simulink model "EvPowertrainController3EMDualRear"  (R2025b)
settings: configuration reference "VehicleFixed10ms" (kept outside this file)
model workspace (MAT data in the model file):
  CtrlVcuAccelPdlBpts = [0 0.8 1]
  CtrlVcuBattPnlty = 10000000
  CtrlVcuBattSOCBpts = [0 20 60 80 100]
  CtrlVcuCnstrntPnltyFctr = 10000000
  CtrlVcuEMPnlty = 100
  CtrlVcuEMTrqSplitGrid = 200
  CtrlVcuFallRate = -500
  CtrlVcuMaxAccelG = 1
  CtrlVcuMaxDecelG = -1.5
  CtrlVcuPwrDeltaPnlty = 50
  CtrlVcuPwrRatePnlty = [25 25 100]
  CtrlVcuRiseRate = 500
  CtrlVcuRoadMuEst = 0.8
  CtrlVcuSftyFctr = 0.9
  CtrlVcuTracPwrErrPnlty = 25
  CtrlVcuTrqVecBrkThresh = 0.01
  CtrlVcuTrqVecIGain = 0
  CtrlVcuTrqVecMinTrq = 25
  CtrlVcuTrqVecPGain = -2000
  CtrlVcuTrqVecSteerThresh = 0.349065850399
  CtrlVcuTrqVecVelThresh = 2.5
  N_P0 = 3
undefined symbols (not defined in the file): CtrlBcuTrlrBrkGain, CtrlVcuEvChrgLmtBpt, CtrlVcuEvRegenBrkCutOff, CtrlVcuEvRegenBrkSpdBpt, CtrlVcuEvSocBpt, eff, EnvGrvty, PlntBrkActrBoreFrnt, PlntBrkActrBoreRear, PlntBrkFrntBias, PlntBrkKinFricCffFrnt, PlntBrkKinFricCffRear, PlntBrkNumPadsFrnt, PlntBrkNumPadsRear, PlntBrkPadMeanRadiusFrnt, PlntBrkPadMeanRadiusRear, PlntBrkPrsFctr, PlntBrkRearBias, PlntDiffrntl2Eff, PlntDiffrntl2Ratio, PlntDiffrntlEff, PlntDiffrntlRatio, PlntEM1EffTbl, PlntEM1Spd, PlntEM1SpdEff, PlntEM1TransEff, PlntEM1TransGearRatio, PlntEM1Trq, PlntEM1TrqEff, PlntEM2EffTbl, PlntEM2Spd, PlntEM2SpdEff, PlntEM2TransEff, PlntEM2TransGearRatio, PlntEM2Trq, PlntEM2TrqEff, PlntEM3EffTbl, PlntEM3Spd, PlntEM3SpdEff, PlntEM3TransEff, PlntEM3TransGearRatio, PlntEM3Trq, PlntEM3TrqEff, PlntEMWhlGearEffFL, PlntEMWhlGearEffRL, PlntEMWhlGearRatioFL, PlntEMWhlGearRatioRL, PlntTransEffSpdBpt, PlntTransEffTbl, PlntTransEffTempBpt, PlntTransEffTrqBpt, PlntTransGearNumVect, PlntTransGearRatioVect, PlntVehCGHgtAxl, PlntVehDstCGFrntAxl, PlntVehDstCGRearAxl, PlntVehMass, PlntWhlLdRadiusFrnt, PlntWhlLdRadiusRear
libraries: simulink x16, autolibutils x2, slpidlib x2
(part 4 of 5)

== system EvPowertrainController3EMDualRear/Energy Management/Calculate Average EMSpd and Wheel Torque Curves for Front and Rear Axles/3EM Dual Rear/EMTrq2WhlTrqRear/Single Speed Transmission ==
  EMTrqCmd : Inport
  EMSpd : Inport  Port=2
  Divide2 : Product  Inputs=**
  Dual EMs : Gain  Gain=2
  Gain3 : Gain  Gain=PlntEMWhlGearRatioRL*PlntEM2TransGearRatio
  Gear Eta : Subsystem
  WhlMotTrq : Outport  VectorParamsAs1DForOutWhenUnconnected=off
  wires:
  Gear Eta/1(eta) -> Divide2/1
  EMTrqCmd/1 -> Dual EMs/1
  EMSpd/1 -> Gear Eta/1(SpdIn)
  Divide2/1 -> WhlMotTrq/1
  Gain3/1 -> Divide2/2
  Dual EMs/1 -> Gain3/1, Gear Eta/2(TrqIn)

== system EvPowertrainController3EMDualRear/Energy Management/Calculate Average EMSpd and Wheel Torque Curves for Front and Rear Axles/3EM Dual Rear/EMTrq2WhlTrqRear/Transmission ==
  Gear : Inport
  EMTrqCmd : Inport  Port=2
  EMSpd : Inport  Port=3
  Diff Eta : Subsystem
  Divide : Product  Inputs=**
  Divide1 : Product  Inputs=**
  Divide2 : Product  Inputs=**
  Divide3 : Product  Inputs=*/
  Gain : Gain  Gain=PlntDiffrntl2Ratio
  Gear ratio look up : LookupNDDirect  NumberOfTableDimensions=1  Table=PlntTransGearRatioVect
  Trans Eta : Subsystem
  WhlMotTrq : Outport  VectorParamsAs1DForOutWhenUnconnected=off
  wires:
  EMSpd/1 -> Trans Eta/2(SpdIn), [Spd]
  EMTrqCmd/1 -> Trans Eta/1(TrqIn), Divide/2
  Divide3/1 -> Diff Eta/1(SpdIn)
  [Spd] -> Divide3/1
  Diff Eta/1(eta) -> Divide2/1
  Divide2/1 -> WhlMotTrq/1
  Divide1/1 -> Gain/1, Diff Eta/2(TrqIn)
  Trans Eta/1(eta) -> Divide1/1
  Gear/1 -> Gear ratio look up/1, Trans Eta/3(Gear)
  Divide/1 -> Divide1/2
  Gear ratio look up/1 -> Divide/1, Divide3/2
  Gain/1 -> Divide2/2

== system EvPowertrainController3EMDualRear/Energy Management/Calculate Average EMSpd and Wheel Torque Curves for Front and Rear Axles/4EM/EMTrq2WhlTrqFrnt/Single Speed Transmission ==
  EMTrqCmd : Inport
  EMSpd : Inport  Port=2
  Divide2 : Product  Inputs=**
  Dual EMs : Gain  Gain=2
  Gain3 : Gain  Gain=PlntEMWhlGearRatioFL*PlntEM1TransGearRatio
  Gear Eta : Subsystem
  WhlMotTrq : Outport  VectorParamsAs1DForOutWhenUnconnected=off
  wires:
  Gain3/1 -> Divide2/2
  Divide2/1 -> WhlMotTrq/1
  EMSpd/1 -> Gear Eta/1(SpdIn)
  EMTrqCmd/1 -> Dual EMs/1
  Gear Eta/1(eta) -> Divide2/1
  Dual EMs/1 -> Gear Eta/2(TrqIn), Gain3/1

== system EvPowertrainController3EMDualRear/Energy Management/Calculate Average EMSpd and Wheel Torque Curves for Front and Rear Axles/4EM/EMTrq2WhlTrqFrnt/Transmission ==
  Gear : Inport
  EMTrqCmd : Inport  Port=2
  EMSpd : Inport  Port=3
  Diff Eta : Subsystem
  Divide : Product  Inputs=**
  Divide1 : Product  Inputs=**
  Divide2 : Product  Inputs=**
  Divide3 : Product  Inputs=*/
  Gain : Gain  Gain=PlntDiffrntlRatio
  Gear ratio look up : LookupNDDirect  NumberOfTableDimensions=1  Table=PlntTransGearRatioVect
  Trans Eta : Subsystem
  WhlMotTrq : Outport  VectorParamsAs1DForOutWhenUnconnected=off
  wires:
  EMSpd/1 -> Trans Eta/2(SpdIn), [Spd]
  EMTrqCmd/1 -> Trans Eta/1(TrqIn), Divide/2
  Divide3/1 -> Diff Eta/1(SpdIn)
  [Spd] -> Divide3/1
  Diff Eta/1(eta) -> Divide2/1
  Divide2/1 -> WhlMotTrq/1
  Divide1/1 -> Gain/1, Diff Eta/2(TrqIn)
  Trans Eta/1(eta) -> Divide1/1
  Gear/1 -> Gear ratio look up/1, Trans Eta/3(Gear)
  Divide/1 -> Divide1/2
  Gear ratio look up/1 -> Divide/1, Divide3/2
  Gain/1 -> Divide2/2

== system EvPowertrainController3EMDualRear/Energy Management/Calculate Average EMSpd and Wheel Torque Curves for Front and Rear Axles/4EM/EMTrq2WhlTrqRear/Single Speed Transmission ==
  EMTrqCmd : Inport
  EMSpd : Inport  Port=2
  Divide2 : Product  Inputs=**
  Dual EMs : Gain  Gain=2
  Gain3 : Gain  Gain=PlntEMWhlGearRatioRL*PlntEM3TransGearRatio
  Gear Eta : Subsystem
  WhlMotTrq : Outport  VectorParamsAs1DForOutWhenUnconnected=off
  wires:
  Gain3/1 -> Divide2/2
  Divide2/1 -> WhlMotTrq/1
  EMSpd/1 -> Gear Eta/1(SpdIn)
  EMTrqCmd/1 -> Dual EMs/1
  Gear Eta/1(eta) -> Divide2/1
  Dual EMs/1 -> Gear Eta/2(TrqIn), Gain3/1

== system EvPowertrainController3EMDualRear/Energy Management/Calculate Average EMSpd and Wheel Torque Curves for Front and Rear Axles/4EM/EMTrq2WhlTrqRear/Transmission ==
  Gear : Inport
  EMTrqCmd : Inport  Port=2
  EMSpd : Inport  Port=3
  Diff Eta : Subsystem
  Divide : Product  Inputs=**
  Divide1 : Product  Inputs=**
  Divide2 : Product  Inputs=**
  Divide3 : Product  Inputs=*/
  Gain : Gain  Gain=PlntDiffrntl2Ratio
  Gear ratio look up : LookupNDDirect  NumberOfTableDimensions=1  Table=PlntTransGearRatioVect
  Trans Eta : Subsystem
  WhlMotTrq : Outport  VectorParamsAs1DForOutWhenUnconnected=off
  wires:
  Gain/1 -> Divide2/2
  Gear ratio look up/1 -> Divide3/2, Divide/1
  Divide/1 -> Divide1/2
  Gear/1 -> Trans Eta/3(Gear), Gear ratio look up/1
  Trans Eta/1(eta) -> Divide1/1
  Divide1/1 -> Diff Eta/2(TrqIn), Gain/1
  Divide2/1 -> WhlMotTrq/1
  Diff Eta/1(eta) -> Divide2/1
  [Spd] -> Divide3/1
  Divide3/1 -> Diff Eta/1(SpdIn)
  EMTrqCmd/1 -> Divide/2, Trans Eta/1(TrqIn)
  EMSpd/1 -> [Spd], Trans Eta/2(SpdIn)

== system EvPowertrainController3EMDualRear/Energy Management/Control Domain /Front Axle EM Torque Vector/2EM or 3EM Dual Rear/Diff Eta ==
  note: Pwr >= 0, v = 1
      | Pwr < 0, v= -1
  SpdIn : Inport
  TrqIn : Inport  Port=2
  Constant : Constant  Value=PlntDiffrntlEff*PlntEM1TransEff
  Constant1 : Constant  SampleTime=-1
  Constant2 : Constant  Value=-1  SampleTime=-1
  Math Function1 : Math  Operator=pow  SignedPower=on  OutputSignalType=real
  Product1 : Product
  Switch2 : Switch  SaturateOnIntegerOverflow=off  InputSameDT=off
  eta : Outport  VectorParamsAs1DForOutWhenUnconnected=off
  wires:
  TrqIn/1 -> Product1/1
  Math Function1/1 -> eta/1
  Switch2/1 -> Math Function1/2
  Product1/1 -> Switch2/2
  Constant1/1 -> Switch2/1
  Constant2/1 -> Switch2/3
  Constant/1 -> Math Function1/1
  SpdIn/1 -> Product1/2

== system EvPowertrainController3EMDualRear/Energy Management/Control Domain /Front Axle EM Torque Vector/3EM Dual Front or 4EM/Gear Eta ==
  note: Pwr >= 0, v = 1
      | Pwr < 0, v= -1
  SpdIn : Inport
  TrqIn : Inport  Port=2
  Constant : Constant  Value=PlntEMWhlGearEffFL*PlntEM1TransEff
  Constant1 : Constant  SampleTime=-1
  Constant2 : Constant  Value=-1  SampleTime=-1
  Math Function1 : Math  Operator=pow  SignedPower=on  OutputSignalType=real
  Product1 : Product
  Switch2 : Switch  SaturateOnIntegerOverflow=off  InputSameDT=off
  eta : Outport  VectorParamsAs1DForOutWhenUnconnected=off
  wires:
  TrqIn/1 -> Product1/1
  Math Function1/1 -> eta/1
  Switch2/1 -> Math Function1/2
  Product1/1 -> Switch2/2
  Constant1/1 -> Switch2/1
  Constant2/1 -> Switch2/3
  Constant/1 -> Math Function1/1
  SpdIn/1 -> Product1/2

== system EvPowertrainController3EMDualRear/Energy Management/Control Domain /Rear Axle EM Torque Vector/2EM/Diff Eta ==
  note: Pwr >= 0, v = 1
      | Pwr < 0, v= -1
  SpdIn : Inport
  TrqIn : Inport  Port=2
  Constant : Constant  Value=PlntDiffrntl2Eff*PlntEM2TransEff
  Constant1 : Constant  SampleTime=-1
  Constant2 : Constant  Value=-1  SampleTime=-1
  Math Function1 : Math  Operator=pow  SignedPower=on  OutputSignalType=real
  Product1 : Product
  Switch2 : Switch  SaturateOnIntegerOverflow=off  InputSameDT=off
  eta : Outport  VectorParamsAs1DForOutWhenUnconnected=off
  wires:
  SpdIn/1 -> Product1/2
  Constant/1 -> Math Function1/1
  Constant2/1 -> Switch2/3
  Constant1/1 -> Switch2/1
  Product1/1 -> Switch2/2
  Switch2/1 -> Math Function1/2
  Math Function1/1 -> eta/1
  TrqIn/1 -> Product1/1

== system EvPowertrainController3EMDualRear/Energy Management/Control Domain /Rear Axle EM Torque Vector/3EM Dual Front/Diff Eta ==
  note: Pwr >= 0, v = 1
      | Pwr < 0, v= -1
  SpdIn : Inport
  TrqIn : Inport  Port=2
  Constant : Constant  Value=PlntDiffrntl2Eff*PlntEM3TransEff
  Constant1 : Constant  SampleTime=-1
  Constant2 : Constant  Value=-1  SampleTime=-1
  Math Function1 : Math  Operator=pow  SignedPower=on  OutputSignalType=real
  Product1 : Product
  Switch2 : Switch  SaturateOnIntegerOverflow=off  InputSameDT=off
  eta : Outport  VectorParamsAs1DForOutWhenUnconnected=off
  wires:
  TrqIn/1 -> Product1/1
  Math Function1/1 -> eta/1
  Switch2/1 -> Math Function1/2
  Product1/1 -> Switch2/2
  Constant1/1 -> Switch2/1
  Constant2/1 -> Switch2/3
  Constant/1 -> Math Function1/1
  SpdIn/1 -> Product1/2

== system EvPowertrainController3EMDualRear/Energy Management/Control Domain /Rear Axle EM Torque Vector/3EM Dual Rear or 4EM/Gear Eta ==
  note: Pwr >= 0, v = 1
      | Pwr < 0, v= -1
  SpdIn : Inport
  TrqIn : Inport  Port=2
  Constant : Constant  Value=PlntEMWhlGearEffRL*PlntEM3TransEff
  Constant1 : Constant  SampleTime=-1
  Constant2 : Constant  Value=-1  SampleTime=-1
  Math Function1 : Math  Operator=pow  SignedPower=on  OutputSignalType=real
  Product1 : Product
  Switch2 : Switch  SaturateOnIntegerOverflow=off  InputSameDT=off
  eta : Outport  VectorParamsAs1DForOutWhenUnconnected=off
  wires:
  SpdIn/1 -> Product1/2
  Constant/1 -> Math Function1/1
  Constant2/1 -> Switch2/3
  Constant1/1 -> Switch2/1
  Product1/1 -> Switch2/2
  Switch2/1 -> Math Function1/2
  Math Function1/1 -> eta/1
  TrqIn/1 -> Product1/1

== system EvPowertrainController3EMDualRear/Energy Management/Powertrain Constraints /Battery Constraint/Electrical Current/DC-DC Eta ==
  In : Inport
  DC-DC Eta : Subsystem  VariantControl=1
  No DC-DC : Subsystem  VariantControl=0
  Out : Outport  VectorParamsAs1DForOutWhenUnconnected=off

== system EvPowertrainController3EMDualRear/Energy Management/Powertrain Constraints /EM Constraint Front/Tabular Power Loss Data/2EM or 3EM Dual Rear ==
  note: Pelec_req = Pmech_req*Eff^k,
      | k = -1 if Motoring >= 0,
      | k = 1 if Generating < 0
  note: Check if Motoring
      | or Generating
  EMAvgSpdVec : Inport
  WhlEMTrqSatVec : Inport  Port=2
  Abs : Abs  SaturateOnIntegerOverflow=off
  Abs1 : Abs  SaturateOnIntegerOverflow=off
  Constant1 : Constant  Value=-1  SampleTime=-1
  Constant2 : Constant  SampleTime=-1
  Eff Map : Lookup_n-D  BreakpointsForDimension1=PlntEM1SpdEff  BreakpointsForDimension2=PlntEM1TrqEff  BeginIndexSearchUsingPreviousIndexResult=on  Table=PlntEM1EffTbl  ExtrapMethod=Clip  UseLastTableValue=on  InternalRulePriority=Speed  OutDataTypeStr=Inherit: Inherit from 'Table data'  RndMeth=Simplest
      settings: InputPortMap=u0,u1
  Gain2 : Gain  Gain=1/100
  Math Function1 : Math  Operator=pow  SignedPower=on  OutputSignalType=real
  Product1 : Product
  Product4 : Product
  Switch2 : Switch  SaturateOnIntegerOverflow=off  InputSameDT=off
  WhlTrq2EMTrq : Subsystem  VariantControl=2EM or 3EMDualFront
  EMPwrElecVec : Outport  VectorParamsAs1DForOutWhenUnconnected=off
  wires:
  WhlEMTrqSatVec/1 -> WhlTrq2EMTrq/2(WhlTrqCmd)
  EMAvgSpdVec/1 -> WhlTrq2EMTrq/1(EMSpd), Product1/1, Abs/1
  Eff Map/1 -> Gain2/1
  Abs1/1 -> Eff Map/2
  Abs/1 -> Eff Map/1
  Gain2/1 -> Math Function1/1
  Constant2/1 -> Switch2/3
  Constant1/1 -> Switch2/1
  Product1/1 -> Switch2/2, Product4/1
  Switch2/1 -> Math Function1/2
  Math Function1/1 -> Product4/2
  Product4/1 -> EMPwrElecVec/1
  WhlTrq2EMTrq/1(EMTrq) -> Abs1/1, Product1/2

== system EvPowertrainController3EMDualRear/Energy Management/Powertrain Constraints /EM Constraint Front/Tabular Power Loss Data/3EM Dual Front or 4EM ==
  note: Check if Motoring
      | or Generating
  note: Pelec_req = Pmech_req*Eff^k,
      | k = -1 if Motoring >= 0,
      | k = 1 if Generating < 0
  EMAvgSpdVec : Inport
  WhlEMTrqSatVec : Inport  Port=2
  Abs : Abs  SaturateOnIntegerOverflow=off
  Abs1 : Abs  SaturateOnIntegerOverflow=off
  Constant1 : Constant  Value=-1  SampleTime=-1
  Constant2 : Constant  SampleTime=-1
  Dual EMs : Gain  Gain=2
  Eff Map : Lookup_n-D  BreakpointsForDimension1=PlntEM1SpdEff  BreakpointsForDimension2=PlntEM1TrqEff  BeginIndexSearchUsingPreviousIndexResult=on  Table=PlntEM1EffTbl  ExtrapMethod=Clip  UseLastTableValue=on  InternalRulePriority=Speed  OutDataTypeStr=Inherit: Inherit from 'Table data'  RndMeth=Simplest
      settings: InputPortMap=u0,u1
  Gain2 : Gain  Gain=1/100
  Math Function1 : Math  Operator=pow  SignedPower=on  OutputSignalType=real
  Product1 : Product
  Product4 : Product
  Switch2 : Switch  SaturateOnIntegerOverflow=off  InputSameDT=off
  WhlTrq2EMTrq : Subsystem  VariantControl=3EMDualRear or 4EM
  EMPwrElecVec : Outport  VectorParamsAs1DForOutWhenUnconnected=off
  wires:
  WhlTrq2EMTrq/1(EMTrq) -> Product1/2, Abs1/1
  Product4/1 -> Dual EMs/1
  Math Function1/1 -> Product4/2
  Switch2/1 -> Math Function1/2
  Product1/1 -> Product4/1, Switch2/2
  Constant1/1 -> Switch2/1
  Constant2/1 -> Switch2/3
  Gain2/1 -> Math Function1/1
  Abs/1 -> Eff Map/1
  Abs1/1 -> Eff Map/2
  Eff Map/1 -> Gain2/1
  EMAvgSpdVec/1 -> WhlTrq2EMTrq/1(EMSpd), Abs/1, Product1/1
  WhlEMTrqSatVec/1 -> WhlTrq2EMTrq/2(WhlTrqCmd)
  Dual EMs/1 -> EMPwrElecVec/1

== system EvPowertrainController3EMDualRear/Energy Management/Powertrain Constraints /EM Constraint Front/Wheel Torque Saturation for Max g Rates/Wheel Torque Limit at Max g Rates ==
  note: Braking sign convention
  Constant6 : Constant  Value=CtrlVcuMaxDecelG  SampleTime=-1
  Constant7 : Constant  Value=CtrlVcuMaxAccelG  SampleTime=-1
  Gain : Gain  Gain=-1
  Wheel Torque at Max Acceleration Rate : Subsystem  VariantControl=tractorVariant==3
  Wheel Torque at Max Deceleration Rate : Subsystem  VariantControl=tractorVariant==3
  WhlTrqLmt_Accel : Outport
  WhlTrqLmt_Brk : Outport  Port=2
  wires:
  Constant6/1 -> Wheel Torque at Max Deceleration Rate/1(MaxAcc)
  Constant7/1 -> Wheel Torque at Max Acceleration Rate/1(MaxAcc)
  Wheel Torque at Max Acceleration Rate/1(WhlTrqLmt) -> WhlTrqLmt_Accel/1
  Wheel Torque at Max Deceleration Rate/1(WhlTrqLmt) -> Gain/1
  Gain/1 -> WhlTrqLmt_Brk/1

== system EvPowertrainController3EMDualRear/Energy Management/Powertrain Constraints /EM Constraint Rear/Tabular Power Loss Data/2EM ==
  note: Pelec_req = Pmech_req*Eff^k,
      | k = -1 if Motoring >= 0,
      | k = 1 if Generating < 0
  note: Check if Motoring
      | or Generating
  EMAvgSpdVec : Inport
  WhlEMTrqSatVec : Inport  Port=2
  Abs : Abs  SaturateOnIntegerOverflow=off
  Abs1 : Abs  SaturateOnIntegerOverflow=off
  Constant1 : Constant  Value=-1  SampleTime=-1
  Constant2 : Constant  SampleTime=-1
  Eff Map : Lookup_n-D  BreakpointsForDimension1=PlntEM2SpdEff  BreakpointsForDimension2=PlntEM2TrqEff  BeginIndexSearchUsingPreviousIndexResult=on  Table=PlntEM2EffTbl  ExtrapMethod=Clip  UseLastTableValue=on  InternalRulePriority=Speed  OutDataTypeStr=Inherit: Inherit from 'Table data'  RndMeth=Simplest
      settings: InputPortMap=u0,u1
  Gain2 : Gain  Gain=1/100
  Math Function1 : Math  Operator=pow  SignedPower=on  OutputSignalType=real
  Product1 : Product
  Product4 : Product
  Switch2 : Switch  SaturateOnIntegerOverflow=off  InputSameDT=off
  WhlTrq2EMTrq : Subsystem  VariantControl=2EM or 3EMDualFront
  EMPwrElecVec : Outport  VectorParamsAs1DForOutWhenUnconnected=off
  wires:
  WhlEMTrqSatVec/1 -> WhlTrq2EMTrq/2(WhlTrqCmd)
  EMAvgSpdVec/1 -> WhlTrq2EMTrq/1(EMSpd), Product1/1, Abs/1
  Eff Map/1 -> Gain2/1
  Abs1/1 -> Eff Map/2
  Abs/1 -> Eff Map/1
  Gain2/1 -> Math Function1/1
  Constant2/1 -> Switch2/3
  Constant1/1 -> Switch2/1
  Product1/1 -> Switch2/2, Product4/1
  Switch2/1 -> Math Function1/2
  Math Function1/1 -> Product4/2
  Product4/1 -> EMPwrElecVec/1
  WhlTrq2EMTrq/1(EMTrq) -> Abs1/1, Product1/2

== system EvPowertrainController3EMDualRear/Energy Management/Powertrain Constraints /EM Constraint Rear/Tabular Power Loss Data/3EM Dual Front ==
  note: Check if Motoring
      | or Generating
  note: Pelec_req = Pmech_req*Eff^k,
      | k = -1 if Motoring >= 0,
      | k = 1 if Generating < 0
  EMAvgSpdVec : Inport
  WhlEMTrqSatVec : Inport  Port=2
  Abs : Abs  SaturateOnIntegerOverflow=off
  Abs1 : Abs  SaturateOnIntegerOverflow=off
  Constant1 : Constant  Value=-1  SampleTime=-1
  Constant2 : Constant  SampleTime=-1
  Eff Map : Lookup_n-D  BreakpointsForDimension1=PlntEM3SpdEff  BreakpointsForDimension2=PlntEM3TrqEff  BeginIndexSearchUsingPreviousIndexResult=on  Table=PlntEM3EffTbl  ExtrapMethod=Clip  UseLastTableValue=on  InternalRulePriority=Speed  OutDataTypeStr=Inherit: Inherit from 'Table data'  RndMeth=Simplest
      settings: InputPortMap=u0,u1
  Gain2 : Gain  Gain=1/100
  Math Function1 : Math  Operator=pow  SignedPower=on  OutputSignalType=real
  Product1 : Product
  Product4 : Product
  Switch2 : Switch  SaturateOnIntegerOverflow=off  InputSameDT=off
  WhlTrq2EMTrq : Subsystem  VariantControl=2EM or 3EMDualFront
  EMPwrElecVec : Outport  VectorParamsAs1DForOutWhenUnconnected=off
  wires:
  WhlTrq2EMTrq/1(EMTrq) -> Product1/2, Abs1/1
  Product4/1 -> EMPwrElecVec/1
  Math Function1/1 -> Product4/2
  Switch2/1 -> Math Function1/2
  Product1/1 -> Product4/1, Switch2/2
  Constant1/1 -> Switch2/1
  Constant2/1 -> Switch2/3
  Gain2/1 -> Math Function1/1
  Abs/1 -> Eff Map/1
  Abs1/1 -> Eff Map/2
  Eff Map/1 -> Gain2/1
  EMAvgSpdVec/1 -> Abs/1, Product1/1, WhlTrq2EMTrq/1(EMSpd)
  WhlEMTrqSatVec/1 -> WhlTrq2EMTrq/2(WhlTrqCmd)

== system EvPowertrainController3EMDualRear/Energy Management/Powertrain Constraints /EM Constraint Rear/Tabular Power Loss Data/3EM Dual Rear or 4EM ==
  note: Check if Motoring
      | or Generating
  note: Pelec_req = Pmech_req*Eff^k,
      | k = -1 if Motoring >= 0,
      | k = 1 if Generating < 0
  EMAvgSpdVec : Inport
  WhlEMTrqSatVec : Inport  Port=2
  Abs : Abs  SaturateOnIntegerOverflow=off
  Abs1 : Abs  SaturateOnIntegerOverflow=off
  Constant1 : Constant  Value=-1  SampleTime=-1
  Constant2 : Constant  SampleTime=-1
  Dual EMs : Gain  Gain=2
  Eff Map : Lookup_n-D  BreakpointsForDimension1=PlntEM3SpdEff  BreakpointsForDimension2=PlntEM3TrqEff  BeginIndexSearchUsingPreviousIndexResult=on  Table=PlntEM3EffTbl  ExtrapMethod=Clip  UseLastTableValue=on  InternalRulePriority=Speed  OutDataTypeStr=Inherit: Inherit from 'Table data'  RndMeth=Simplest
      settings: InputPortMap=u0,u1
  Gain2 : Gain  Gain=1/100
  Math Function1 : Math  Operator=pow  SignedPower=on  OutputSignalType=real
  Product1 : Product
  Product4 : Product
  Switch2 : Switch  SaturateOnIntegerOverflow=off  InputSameDT=off
  WhlTrq2EMTrq : Subsystem  VariantControl=3EMDualRear or 4EM
  EMPwrElecVec : Outport  VectorParamsAs1DForOutWhenUnconnected=off
  wires:
  WhlTrq2EMTrq/1(EMTrq) -> Product1/2, Abs1/1
  Product4/1 -> Dual EMs/1
  Math Function1/1 -> Product4/2
  Switch2/1 -> Math Function1/2
  Product1/1 -> Product4/1, Switch2/2
  Constant1/1 -> Switch2/1
  Constant2/1 -> Switch2/3
  Gain2/1 -> Math Function1/1
  Abs/1 -> Eff Map/1
  Abs1/1 -> Eff Map/2
  Eff Map/1 -> Gain2/1
  EMAvgSpdVec/1 -> WhlTrq2EMTrq/1(EMSpd), Abs/1, Product1/1
  WhlEMTrqSatVec/1 -> WhlTrq2EMTrq/2(WhlTrqCmd)
  Dual EMs/1 -> EMPwrElecVec/1

== system EvPowertrainController3EMDualRear/Energy Management/Powertrain Constraints /EM Constraint Rear/Wheel Torque Saturation for Max g Rates/Wheel Torque Limit at Max g Rates ==
  note: Braking sign convention
  Constant6 : Constant  Value=CtrlVcuMaxDecelG  SampleTime=-1
  Constant7 : Constant  Value=CtrlVcuMaxAccelG  SampleTime=-1
  Gain : Gain  Gain=-1
  Wheel Torque at Max Acceleration Rate : Subsystem  VariantControl=tractorVariant==3
  Wheel Torque at Max Deceleration Rate : Subsystem  VariantControl=tractorVariant==3
  WhlTrqLmt_Accel : Outport
  WhlTrqLmt_Brk : Outport  Port=2
  wires:
  Constant6/1 -> Wheel Torque at Max Deceleration Rate/1(MaxAcc)
  Constant7/1 -> Wheel Torque at Max Acceleration Rate/1(MaxAcc)
  Wheel Torque at Max Acceleration Rate/1(WhlTrqLmt) -> WhlTrqLmt_Accel/1
  Wheel Torque at Max Deceleration Rate/1(WhlTrqLmt) -> Gain/1
  Gain/1 -> WhlTrqLmt_Brk/1

== system EvPowertrainController3EMDualRear/Torque Vectoring/3EM/EMTrq/3EMDualFront/3EMDualFront ==
  note: Calculate average speed
      | of EMs on axle
  EMSpd : Inport
  Gain : Gain  Gain=1/2
  Selector : Selector  InputPortWidth=3  IndexOptions=Index vector (dialog)  Indices=[1 2]  OutputSizes=1
  Sum of Elements : Sum  Inputs=+
  EMSpdAvg : Outport
  wires:
  Gain/1 -> EMSpdAvg/1
  Sum of Elements/1 -> Gain/1
  EMSpd/1 -> Selector/1
  Selector/1 -> Sum of Elements/1

== system EvPowertrainController3EMDualRear/Torque Vectoring/3EM/EMTrq/3EMDualRear/3EMDualRear ==
  note: Calculate average speed
      | of EMs on axle
  EMSpd : Inport
  Gain : Gain  Gain=1/2
  Selector : Selector  InputPortWidth=3  IndexOptions=Index vector (dialog)  Indices=[2 3]  OutputSizes=1
  Sum of Elements : Sum  Inputs=+
  EMSpdAvg : Outport
  wires:
  Selector/1 -> Sum of Elements/1
  EMSpd/1 -> Selector/1
  Sum of Elements/1 -> Gain/1
  Gain/1 -> EMSpdAvg/1

== system EvPowertrainController3EMDualRear/Torque Vectoring/4EM/EMTrq/Dual Front/3EMDualFrnt ==
  note: Calculate average speed
      | of EMs on axle
  EMSpd : Inport
  Gain : Gain  Gain=1/2
  Selector : Selector  InputPortWidth=4  IndexOptions=Index vector (dialog)  Indices=[1 2]  OutputSizes=1
  Sum of Elements : Sum  Inputs=+
  EMSpdAvg : Outport
  wires:
  Selector/1 -> Sum of Elements/1
  EMSpd/1 -> Selector/1
  Sum of Elements/1 -> Gain/1
  Gain/1 -> EMSpdAvg/1

== system EvPowertrainController3EMDualRear/Torque Vectoring/4EM/EMTrq/Dual Rear/3EMDualRear ==
  note: Calculate average speed
      | of EMs on axle
  EMSpd : Inport
  Gain : Gain  Gain=1/2
  Selector : Selector  InputPortWidth=4  IndexOptions=Index vector (dialog)  Indices=[3 4]  OutputSizes=1
  Sum of Elements : Sum  Inputs=+
  EMSpdAvg : Outport
  wires:
  Gain/1 -> EMSpdAvg/1
  Sum of Elements/1 -> Gain/1
  EMSpd/1 -> Selector/1
  Selector/1 -> Sum of Elements/1

== system EvPowertrainController3EMDualRear/Accel Pedal to Traction Wheel Torque Request/EM2WhlTrq/2EM/EMTrq2WhlTrqFrnt/Single Speed Transmission/Diff Eta ==
  note: Pwr >= 0, v = 1
      | Pwr < 0, v= -1
  SpdIn : Inport
  TrqIn : Inport  Port=2
  Constant : Constant  Value=PlntDiffrntlEff*PlntEM1TransEff
  Constant1 : Constant  SampleTime=-1
  Constant2 : Constant  Value=-1  SampleTime=-1
  Math Function1 : Math  Operator=pow  SignedPower=on  OutputSignalType=real
  Product1 : Product
  Switch2 : Switch  SaturateOnIntegerOverflow=off  InputSameDT=off
  eta : Outport  VectorParamsAs1DForOutWhenUnconnected=off
  wires:
  SpdIn/1 -> Product1/2
  Constant/1 -> Math Function1/1
  Constant2/1 -> Switch2/3
  Constant1/1 -> Switch2/1
  Product1/1 -> Switch2/2
  Switch2/1 -> Math Function1/2
  Math Function1/1 -> eta/1
  TrqIn/1 -> Product1/1

== system EvPowertrainController3EMDualRear/Accel Pedal to Traction Wheel Torque Request/EM2WhlTrq/2EM/EMTrq2WhlTrqFrnt/Transmission/Diff Eta ==
  SpdIn : Inport
  TrqIn : Inport  Port=2
  Constant : Constant  Value=PlntDiffrntlEff
  Constant1 : Constant  SampleTime=-1
  Constant2 : Constant  Value=-1  SampleTime=-1
  Math Function1 : Math  Operator=pow  SignedPower=on  OutputSignalType=real
  Product1 : Product
  Switch2 : Switch  SaturateOnIntegerOverflow=off  InputSameDT=off
  eta : Outport  VectorParamsAs1DForOutWhenUnconnected=off
  wires:
  SpdIn/1 -> Product1/2
  Constant/1 -> Math Function1/1
  Constant2/1 -> Switch2/3
  Constant1/1 -> Switch2/1
  Product1/1 -> Switch2/2
  Switch2/1 -> Math Function1/2
  Math Function1/1 -> eta/1
  TrqIn/1 -> Product1/1

== system EvPowertrainController3EMDualRear/Accel Pedal to Traction Wheel Torque Request/EM2WhlTrq/2EM/EMTrq2WhlTrqFrnt/Transmission/Trans Eta ==
  TrqIn : Inport
  SpdIn : Inport  Port=2
  Gear : Inport  Port=3
  Abs1 : Abs  SaturateOnIntegerOverflow=off
  Constant : Constant  Value=PlntTransEffTempBpt(1)
  Constant1 : Constant  SampleTime=-1
  Constant2 : Constant  Value=-1  SampleTime=-1
  Eta 4D : Lookup_n-D  NumberOfTableDimensions=4  LookupTableObject=''  BreakpointsForDimension1=PlntTransEffTrqBpt  BreakpointsForDimension2=PlntTransEffSpdBpt  BreakpointsForDimension3=PlntTransGearNumVect  BreakpointsForDimension4=PlntTransEffTempBpt  Table=PlntTransEffTbl  ExtrapMethod=Clip  InternalRulePriority=Speed  RndMeth=Simplest
      settings: InputPortMap=u0,u1,u2,u3
  Math Function1 : Math  Operator=pow  SignedPower=on  OutputSignalType=real
  Product1 : Product
  Switch2 : Switch  SaturateOnIntegerOverflow=off  InputSameDT=off
  eta : Outport  VectorParamsAs1DForOutWhenUnconnected=off
  wires:
  TrqIn/1 -> Product1/1, Abs1/1
  Math Function1/1 -> eta/1
  Abs1/1 -> Eta 4D/1
  Switch2/1 -> Math Function1/2
  Product1/1 -> Switch2/2
  Constant1/1 -> Switch2/1
  Constant2/1 -> Switch2/3
  Eta 4D/1 -> Math Function1/1
  SpdIn/1 -> Product1/2, Eta 4D/2
  Gear/1 -> Eta 4D/3
  Constant/1 -> Eta 4D/4

== system EvPowertrainController3EMDualRear/Accel Pedal to Traction Wheel Torque Request/EM2WhlTrq/2EM/EMTrq2WhlTrqRear/Single Speed Transmission/Diff Eta ==
  note: Pwr >= 0, v = 1
      | Pwr < 0, v= -1
  SpdIn : Inport
  TrqIn : Inport  Port=2
  Constant : Constant  Value=PlntDiffrntl2Eff*PlntEM2TransEff
  Constant1 : Constant  SampleTime=-1
  Constant2 : Constant  Value=-1  SampleTime=-1
  Math Function1 : Math  Operator=pow  SignedPower=on  OutputSignalType=real
  Product1 : Product
  Switch2 : Switch  SaturateOnIntegerOverflow=off  InputSameDT=off
  eta : Outport  VectorParamsAs1DForOutWhenUnconnected=off
  wires:
  SpdIn/1 -> Product1/2
  Constant/1 -> Math Function1/1
  Constant2/1 -> Switch2/3
  Constant1/1 -> Switch2/1
  Product1/1 -> Switch2/2
  Switch2/1 -> Math Function1/2
  Math Function1/1 -> eta/1
  TrqIn/1 -> Product1/1

== system EvPowertrainController3EMDualRear/Accel Pedal to Traction Wheel Torque Request/EM2WhlTrq/2EM/EMTrq2WhlTrqRear/Transmission/Diff Eta ==
  SpdIn : Inport
  TrqIn : Inport  Port=2
  Constant : Constant  Value=PlntDiffrntl2Eff
  Constant1 : Constant  SampleTime=-1
  Constant2 : Constant  Value=-1  SampleTime=-1
  Math Function1 : Math  Operator=pow  SignedPower=on  OutputSignalType=real
  Product1 : Product
  Switch2 : Switch  SaturateOnIntegerOverflow=off  InputSameDT=off
  eta : Outport  VectorParamsAs1DForOutWhenUnconnected=off
  wires:
  TrqIn/1 -> Product1/1
  Math Function1/1 -> eta/1
  Switch2/1 -> Math Function1/2
  Product1/1 -> Switch2/2
  Constant1/1 -> Switch2/1
  Constant2/1 -> Switch2/3
  Constant/1 -> Math Function1/1
  SpdIn/1 -> Product1/2

== system EvPowertrainController3EMDualRear/Accel Pedal to Traction Wheel Torque Request/EM2WhlTrq/2EM/EMTrq2WhlTrqRear/Transmission/Trans Eta ==
  TrqIn : Inport
  SpdIn : Inport  Port=2
  Gear : Inport  Port=3
  Abs1 : Abs  SaturateOnIntegerOverflow=off
  Constant : Constant  Value=PlntTransEffTempBpt(1)
  Constant1 : Constant  SampleTime=-1
  Constant2 : Constant  Value=-1  SampleTime=-1
  Eta 4D : Lookup_n-D  NumberOfTableDimensions=4  LookupTableObject=''  BreakpointsForDimension1=PlntTransEffTrqBpt  BreakpointsForDimension2=PlntTransEffSpdBpt  BreakpointsForDimension3=PlntTransGearNumVect  BreakpointsForDimension4=PlntTransEffTempBpt  Table=PlntTransEffTbl  ExtrapMethod=Clip  InternalRulePriority=Speed  RndMeth=Simplest
      settings: InputPortMap=u0,u1,u2,u3
  Math Function1 : Math  Operator=pow  SignedPower=on  OutputSignalType=real
  Product1 : Product
  Switch2 : Switch  SaturateOnIntegerOverflow=off  InputSameDT=off
  eta : Outport  VectorParamsAs1DForOutWhenUnconnected=off
  wires:
  Constant/1 -> Eta 4D/4
  Gear/1 -> Eta 4D/3
  SpdIn/1 -> Eta 4D/2, Product1/2
  Eta 4D/1 -> Math Function1/1
  Constant2/1 -> Switch2/3
  Constant1/1 -> Switch2/1
  Product1/1 -> Switch2/2
  Switch2/1 -> Math Function1/2
  Abs1/1 -> Eta 4D/1
  Math Function1/1 -> eta/1
  TrqIn/1 -> Abs1/1, Product1/1

== system EvPowertrainController3EMDualRear/Accel Pedal to Traction Wheel Torque Request/EM2WhlTrq/3EM Dual Front/EMTrq2WhlTrqFrnt/Single Speed Transmission/Gear Eta ==
  note: Pwr >= 0, v = 1
      | Pwr < 0, v= -1
  SpdIn : Inport
  TrqIn : Inport  Port=2
  Constant : Constant  Value=PlntEMWhlGearEffFL*PlntEM1TransEff
  Constant1 : Constant  SampleTime=-1
  Constant2 : Constant  Value=-1  SampleTime=-1
  Math Function1 : Math  Operator=pow  SignedPower=on  OutputSignalType=real
  Product1 : Product
  Switch2 : Switch  SaturateOnIntegerOverflow=off  InputSameDT=off
  eta : Outport  VectorParamsAs1DForOutWhenUnconnected=off
  wires:
  TrqIn/1 -> Product1/1
  Math Function1/1 -> eta/1
  Switch2/1 -> Math Function1/2
  Product1/1 -> Switch2/2
  Constant1/1 -> Switch2/1
  Constant2/1 -> Switch2/3
  Constant/1 -> Math Function1/1
  SpdIn/1 -> Product1/2

== system EvPowertrainController3EMDualRear/Accel Pedal to Traction Wheel Torque Request/EM2WhlTrq/3EM Dual Front/EMTrq2WhlTrqFrnt/Transmission/Diff Eta ==
  SpdIn : Inport
  TrqIn : Inport  Port=2
  Constant : Constant  Value=PlntDiffrntlEff
  Constant1 : Constant  SampleTime=-1
  Constant2 : Constant  Value=-1  SampleTime=-1
  Math Function1 : Math  Operator=pow  SignedPower=on  OutputSignalType=real
  Product1 : Product
  Switch2 : Switch  SaturateOnIntegerOverflow=off  InputSameDT=off
  eta : Outport  VectorParamsAs1DForOutWhenUnconnected=off
  wires:
  TrqIn/1 -> Product1/1
  Math Function1/1 -> eta/1
  Switch2/1 -> Math Function1/2
  Product1/1 -> Switch2/2
  Constant1/1 -> Switch2/1
  Constant2/1 -> Switch2/3
  Constant/1 -> Math Function1/1
  SpdIn/1 -> Product1/2

== system EvPowertrainController3EMDualRear/Accel Pedal to Traction Wheel Torque Request/EM2WhlTrq/3EM Dual Front/EMTrq2WhlTrqFrnt/Transmission/Trans Eta ==
  TrqIn : Inport
  SpdIn : Inport  Port=2
  Gear : Inport  Port=3
  Abs1 : Abs  SaturateOnIntegerOverflow=off
  Constant : Constant  Value=PlntTransEffTempBpt(1)
  Constant1 : Constant  SampleTime=-1
  Constant2 : Constant  Value=-1  SampleTime=-1
  Eta 4D : Lookup_n-D  NumberOfTableDimensions=4  LookupTableObject=''  BreakpointsForDimension1=PlntTransEffTrqBpt  BreakpointsForDimension2=PlntTransEffSpdBpt  BreakpointsForDimension3=PlntTransGearNumVect  BreakpointsForDimension4=PlntTransEffTempBpt  Table=PlntTransEffTbl  ExtrapMethod=Clip  InternalRulePriority=Speed  RndMeth=Simplest
      settings: InputPortMap=u0,u1,u2,u3
  Math Function1 : Math  Operator=pow  SignedPower=on  OutputSignalType=real
  Product1 : Product
  Switch2 : Switch  SaturateOnIntegerOverflow=off  InputSameDT=off
  eta : Outport  VectorParamsAs1DForOutWhenUnconnected=off
  wires:
  Constant/1 -> Eta 4D/4
  Gear/1 -> Eta 4D/3
  SpdIn/1 -> Eta 4D/2, Product1/2
  Eta 4D/1 -> Math Function1/1
  Constant2/1 -> Switch2/3
  Constant1/1 -> Switch2/1
  Product1/1 -> Switch2/2
  Switch2/1 -> Math Function1/2
  Abs1/1 -> Eta 4D/1
  Math Function1/1 -> eta/1
  TrqIn/1 -> Abs1/1, Product1/1

== system EvPowertrainController3EMDualRear/Accel Pedal to Traction Wheel Torque Request/EM2WhlTrq/3EM Dual Front/EMTrq2WhlTrqRear/Single Speed Transmission/Diff Eta ==
  note: Pwr >= 0, v = 1
      | Pwr < 0, v= -1
  SpdIn : Inport
  TrqIn : Inport  Port=2
  Constant : Constant  Value=PlntDiffrntl2Eff*PlntEM3TransEff
  Constant1 : Constant  SampleTime=-1
  Constant2 : Constant  Value=-1  SampleTime=-1
  Math Function1 : Math  Operator=pow  SignedPower=on  OutputSignalType=real
  Product1 : Product
  Switch2 : Switch  SaturateOnIntegerOverflow=off  InputSameDT=off
  eta : Outport  VectorParamsAs1DForOutWhenUnconnected=off
  wires:
  TrqIn/1 -> Product1/1
  Math Function1/1 -> eta/1
  Switch2/1 -> Math Function1/2
  Product1/1 -> Switch2/2
  Constant1/1 -> Switch2/1
  Constant2/1 -> Switch2/3
  Constant/1 -> Math Function1/1
  SpdIn/1 -> Product1/2

== system EvPowertrainController3EMDualRear/Accel Pedal to Traction Wheel Torque Request/EM2WhlTrq/3EM Dual Front/EMTrq2WhlTrqRear/Transmission/Diff Eta ==
  SpdIn : Inport
  TrqIn : Inport  Port=2
  Constant : Constant  Value=PlntDiffrntl2Eff
  Constant1 : Constant  SampleTime=-1
  Constant2 : Constant  Value=-1  SampleTime=-1
  Math Function1 : Math  Operator=pow  SignedPower=on  OutputSignalType=real
  Product1 : Product
  Switch2 : Switch  SaturateOnIntegerOverflow=off  InputSameDT=off
  eta : Outport  VectorParamsAs1DForOutWhenUnconnected=off
  wires:
  SpdIn/1 -> Product1/2
  Constant/1 -> Math Function1/1
  Constant2/1 -> Switch2/3
  Constant1/1 -> Switch2/1
  Product1/1 -> Switch2/2
  Switch2/1 -> Math Function1/2
  Math Function1/1 -> eta/1
  TrqIn/1 -> Product1/1

== system EvPowertrainController3EMDualRear/Accel Pedal to Traction Wheel Torque Request/EM2WhlTrq/3EM Dual Front/EMTrq2WhlTrqRear/Transmission/Trans Eta ==
  TrqIn : Inport
  SpdIn : Inport  Port=2
  Gear : Inport  Port=3
  Abs1 : Abs  SaturateOnIntegerOverflow=off
  Constant : Constant  Value=PlntTransEffTempBpt(1)
  Constant1 : Constant  SampleTime=-1
  Constant2 : Constant  Value=-1  SampleTime=-1
  Eta 4D : Lookup_n-D  NumberOfTableDimensions=4  LookupTableObject=''  BreakpointsForDimension1=PlntTransEffTrqBpt  BreakpointsForDimension2=PlntTransEffSpdBpt  BreakpointsForDimension3=PlntTransGearNumVect  BreakpointsForDimension4=PlntTransEffTempBpt  Table=PlntTransEffTbl  ExtrapMethod=Clip  InternalRulePriority=Speed  RndMeth=Simplest
      settings: InputPortMap=u0,u1,u2,u3
  Math Function1 : Math  Operator=pow  SignedPower=on  OutputSignalType=real
  Product1 : Product
  Switch2 : Switch  SaturateOnIntegerOverflow=off  InputSameDT=off
  eta : Outport  VectorParamsAs1DForOutWhenUnconnected=off
  wires:
  TrqIn/1 -> Product1/1, Abs1/1
  Math Function1/1 -> eta/1
  Abs1/1 -> Eta 4D/1
  Switch2/1 -> Math Function1/2
  Product1/1 -> Switch2/2
  Constant1/1 -> Switch2/1
  Constant2/1 -> Switch2/3
  Eta 4D/1 -> Math Function1/1
  SpdIn/1 -> Product1/2, Eta 4D/2
  Gear/1 -> Eta 4D/3
  Constant/1 -> Eta 4D/4

== system EvPowertrainController3EMDualRear/Accel Pedal to Traction Wheel Torque Request/EM2WhlTrq/3EM Dual Rear/EMTrq2WhlTrqFrnt/Single Speed Transmission/Diff Eta ==
  note: Pwr >= 0, v = 1
      | Pwr < 0, v= -1
  SpdIn : Inport
  TrqIn : Inport  Port=2
  Constant : Constant  Value=PlntDiffrntlEff*PlntEM1TransEff
  Constant1 : Constant  SampleTime=-1
  Constant2 : Constant  Value=-1  SampleTime=-1
  Math Function1 : Math  Operator=pow  SignedPower=on  OutputSignalType=real
  Product1 : Product
  Switch2 : Switch  SaturateOnIntegerOverflow=off  InputSameDT=off
  eta : Outport  VectorParamsAs1DForOutWhenUnconnected=off
  wires:
  SpdIn/1 -> Product1/2
  Constant/1 -> Math Function1/1
  Constant2/1 -> Switch2/3
  Constant1/1 -> Switch2/1
  Product1/1 -> Switch2/2
  Switch2/1 -> Math Function1/2
  Math Function1/1 -> eta/1
  TrqIn/1 -> Product1/1

== system EvPowertrainController3EMDualRear/Accel Pedal to Traction Wheel Torque Request/EM2WhlTrq/3EM Dual Rear/EMTrq2WhlTrqFrnt/Transmission/Diff Eta ==
  SpdIn : Inport
  TrqIn : Inport  Port=2
  Constant : Constant  Value=PlntDiffrntlEff
  Constant1 : Constant  SampleTime=-1
  Constant2 : Constant  Value=-1  SampleTime=-1
  Math Function1 : Math  Operator=pow  SignedPower=on  OutputSignalType=real
  Product1 : Product
  Switch2 : Switch  SaturateOnIntegerOverflow=off  InputSameDT=off
  eta : Outport  VectorParamsAs1DForOutWhenUnconnected=off
  wires:
  SpdIn/1 -> Product1/2
  Constant/1 -> Math Function1/1
  Constant2/1 -> Switch2/3
  Constant1/1 -> Switch2/1
  Product1/1 -> Switch2/2
  Switch2/1 -> Math Function1/2
  Math Function1/1 -> eta/1
  TrqIn/1 -> Product1/1

== system EvPowertrainController3EMDualRear/Accel Pedal to Traction Wheel Torque Request/EM2WhlTrq/3EM Dual Rear/EMTrq2WhlTrqFrnt/Transmission/Trans Eta ==
  TrqIn : Inport
  SpdIn : Inport  Port=2
  Gear : Inport  Port=3
  Abs1 : Abs  SaturateOnIntegerOverflow=off
  Constant : Constant  Value=PlntTransEffTempBpt(1)
  Constant1 : Constant  SampleTime=-1
  Constant2 : Constant  Value=-1  SampleTime=-1
  Eta 4D : Lookup_n-D  NumberOfTableDimensions=4  LookupTableObject=''  BreakpointsForDimension1=PlntTransEffTrqBpt  BreakpointsForDimension2=PlntTransEffSpdBpt  BreakpointsForDimension3=PlntTransGearNumVect  BreakpointsForDimension4=PlntTransEffTempBpt  Table=PlntTransEffTbl  ExtrapMethod=Clip  InternalRulePriority=Speed  RndMeth=Simplest
      settings: InputPortMap=u0,u1,u2,u3
  Math Function1 : Math  Operator=pow  SignedPower=on  OutputSignalType=real
  Product1 : Product
  Switch2 : Switch  SaturateOnIntegerOverflow=off  InputSameDT=off
  eta : Outport  VectorParamsAs1DForOutWhenUnconnected=off
  wires:
  TrqIn/1 -> Product1/1, Abs1/1
  Math Function1/1 -> eta/1
  Abs1/1 -> Eta 4D/1
  Switch2/1 -> Math Function1/2
  Product1/1 -> Switch2/2
  Constant1/1 -> Switch2/1
  Constant2/1 -> Switch2/3
  Eta 4D/1 -> Math Function1/1
  SpdIn/1 -> Product1/2, Eta 4D/2
  Gear/1 -> Eta 4D/3
  Constant/1 -> Eta 4D/4

== system EvPowertrainController3EMDualRear/Accel Pedal to Traction Wheel Torque Request/EM2WhlTrq/3EM Dual Rear/EMTrq2WhlTrqRear/Single Speed Transmission/Gear Eta ==
  note: Pwr >= 0, v = 1
      | Pwr < 0, v= -1
  SpdIn : Inport
  TrqIn : Inport  Port=2
  Constant : Constant  Value=PlntEMWhlGearEffRL*PlntEM2TransEff
  Constant1 : Constant  SampleTime=-1
  Constant2 : Constant  Value=-1  SampleTime=-1
  Math Function1 : Math  Operator=pow  SignedPower=on  OutputSignalType=real
  Product1 : Product
  Switch2 : Switch  SaturateOnIntegerOverflow=off  InputSameDT=off
  eta : Outport  VectorParamsAs1DForOutWhenUnconnected=off
  wires:
  SpdIn/1 -> Product1/2
  Constant/1 -> Math Function1/1
  Constant2/1 -> Switch2/3
  Constant1/1 -> Switch2/1
  Product1/1 -> Switch2/2
  Switch2/1 -> Math Function1/2
  Math Function1/1 -> eta/1
  TrqIn/1 -> Product1/1

== system EvPowertrainController3EMDualRear/Accel Pedal to Traction Wheel Torque Request/EM2WhlTrq/3EM Dual Rear/EMTrq2WhlTrqRear/Transmission/Diff Eta ==
  SpdIn : Inport
  TrqIn : Inport  Port=2
  Constant : Constant  Value=PlntDiffrntl2Eff
  Constant1 : Constant  SampleTime=-1
  Constant2 : Constant  Value=-1  SampleTime=-1
  Math Function1 : Math  Operator=pow  SignedPower=on  OutputSignalType=real
  Product1 : Product
  Switch2 : Switch  SaturateOnIntegerOverflow=off  InputSameDT=off
  eta : Outport  VectorParamsAs1DForOutWhenUnconnected=off
  wires:
  TrqIn/1 -> Product1/1
  Math Function1/1 -> eta/1
  Switch2/1 -> Math Function1/2
  Product1/1 -> Switch2/2
  Constant1/1 -> Switch2/1
  Constant2/1 -> Switch2/3
  Constant/1 -> Math Function1/1
  SpdIn/1 -> Product1/2

== system EvPowertrainController3EMDualRear/Accel Pedal to Traction Wheel Torque Request/EM2WhlTrq/3EM Dual Rear/EMTrq2WhlTrqRear/Transmission/Trans Eta ==
  TrqIn : Inport
  SpdIn : Inport  Port=2
  Gear : Inport  Port=3
  Abs1 : Abs  SaturateOnIntegerOverflow=off
  Constant : Constant  Value=PlntTransEffTempBpt(1)
  Constant1 : Constant  SampleTime=-1
  Constant2 : Constant  Value=-1  SampleTime=-1
  Eta 4D : Lookup_n-D  NumberOfTableDimensions=4  LookupTableObject=''  BreakpointsForDimension1=PlntTransEffTrqBpt  BreakpointsForDimension2=PlntTransEffSpdBpt  BreakpointsForDimension3=PlntTransGearNumVect  BreakpointsForDimension4=PlntTransEffTempBpt  Table=PlntTransEffTbl  ExtrapMethod=Clip  InternalRulePriority=Speed  RndMeth=Simplest
      settings: InputPortMap=u0,u1,u2,u3
  Math Function1 : Math  Operator=pow  SignedPower=on  OutputSignalType=real
  Product1 : Product
  Switch2 : Switch  SaturateOnIntegerOverflow=off  InputSameDT=off
  eta : Outport  VectorParamsAs1DForOutWhenUnconnected=off
  wires:
  Constant/1 -> Eta 4D/4
  Gear/1 -> Eta 4D/3
  SpdIn/1 -> Eta 4D/2, Product1/2
  Eta 4D/1 -> Math Function1/1
  Constant2/1 -> Switch2/3
  Constant1/1 -> Switch2/1
  Product1/1 -> Switch2/2
  Switch2/1 -> Math Function1/2
  Abs1/1 -> Eta 4D/1
  Math Function1/1 -> eta/1
  TrqIn/1 -> Abs1/1, Product1/1

== system EvPowertrainController3EMDualRear/Accel Pedal to Traction Wheel Torque Request/EM2WhlTrq/4EM/EMTrq2WhlTrqFrnt/Single Speed Transmission/Gear Eta ==
  note: Pwr >= 0, v = 1
      | Pwr < 0, v= -1
  SpdIn : Inport
  TrqIn : Inport  Port=2
  Constant : Constant  Value=PlntEMWhlGearEffFL*PlntEM1TransEff
  Constant1 : Constant  SampleTime=-1
  Constant2 : Constant  Value=-1  SampleTime=-1
  Math Function1 : Math  Operator=pow  SignedPower=on  OutputSignalType=real
  Product1 : Product
  Switch2 : Switch  SaturateOnIntegerOverflow=off  InputSameDT=off
  eta : Outport  VectorParamsAs1DForOutWhenUnconnected=off
  wires:
  TrqIn/1 -> Product1/1
  Math Function1/1 -> eta/1
  Switch2/1 -> Math Function1/2
  Product1/1 -> Switch2/2
  Constant1/1 -> Switch2/1
  Constant2/1 -> Switch2/3
  Constant/1 -> Math Function1/1
  SpdIn/1 -> Product1/2

== system EvPowertrainController3EMDualRear/Accel Pedal to Traction Wheel Torque Request/EM2WhlTrq/4EM/EMTrq2WhlTrqFrnt/Transmission/Diff Eta ==
  SpdIn : Inport
  TrqIn : Inport  Port=2
  Constant : Constant  Value=PlntDiffrntlEff
  Constant1 : Constant  SampleTime=-1
  Constant2 : Constant  Value=-1  SampleTime=-1
  Math Function1 : Math  Operator=pow  SignedPower=on  OutputSignalType=real
  Product1 : Product
  Switch2 : Switch  SaturateOnIntegerOverflow=off  InputSameDT=off
  eta : Outport  VectorParamsAs1DForOutWhenUnconnected=off
  wires:
  TrqIn/1 -> Product1/1
  Math Function1/1 -> eta/1
  Switch2/1 -> Math Function1/2
  Product1/1 -> Switch2/2
  Constant1/1 -> Switch2/1
  Constant2/1 -> Switch2/3
  Constant/1 -> Math Function1/1
  SpdIn/1 -> Product1/2

== system EvPowertrainController3EMDualRear/Accel Pedal to Traction Wheel Torque Request/EM2WhlTrq/4EM/EMTrq2WhlTrqFrnt/Transmission/Trans Eta ==
  TrqIn : Inport
  SpdIn : Inport  Port=2
  Gear : Inport  Port=3
  Abs1 : Abs  SaturateOnIntegerOverflow=off
  Constant : Constant  Value=PlntTransEffTempBpt(1)
  Constant1 : Constant  SampleTime=-1
  Constant2 : Constant  Value=-1  SampleTime=-1
  Eta 4D : Lookup_n-D  NumberOfTableDimensions=4  LookupTableObject=''  BreakpointsForDimension1=PlntTransEffTrqBpt  BreakpointsForDimension2=PlntTransEffSpdBpt  BreakpointsForDimension3=PlntTransGearNumVect  BreakpointsForDimension4=PlntTransEffTempBpt  Table=PlntTransEffTbl  ExtrapMethod=Clip  InternalRulePriority=Speed  RndMeth=Simplest
      settings: InputPortMap=u0,u1,u2,u3
  Math Function1 : Math  Operator=pow  SignedPower=on  OutputSignalType=real
  Product1 : Product
  Switch2 : Switch  SaturateOnIntegerOverflow=off  InputSameDT=off
  eta : Outport  VectorParamsAs1DForOutWhenUnconnected=off
  wires:
  Constant/1 -> Eta 4D/4
  Gear/1 -> Eta 4D/3
  SpdIn/1 -> Eta 4D/2, Product1/2
  Eta 4D/1 -> Math Function1/1
  Constant2/1 -> Switch2/3
  Constant1/1 -> Switch2/1
  Product1/1 -> Switch2/2
  Switch2/1 -> Math Function1/2
  Abs1/1 -> Eta 4D/1
  Math Function1/1 -> eta/1
  TrqIn/1 -> Abs1/1, Product1/1

== system EvPowertrainController3EMDualRear/Accel Pedal to Traction Wheel Torque Request/EM2WhlTrq/4EM/EMTrq2WhlTrqRear/Single Speed Transmission/Gear Eta ==
  note: Pwr >= 0, v = 1
      | Pwr < 0, v= -1
  SpdIn : Inport
  TrqIn : Inport  Port=2
  Constant : Constant  Value=PlntEMWhlGearEffRL*PlntEM3TransEff
  Constant1 : Constant  SampleTime=-1
  Constant2 : Constant  Value=-1  SampleTime=-1
  Math Function1 : Math  Operator=pow  SignedPower=on  OutputSignalType=real
  Product1 : Product
  Switch2 : Switch  SaturateOnIntegerOverflow=off  InputSameDT=off
  eta : Outport  VectorParamsAs1DForOutWhenUnconnected=off
  wires:
  TrqIn/1 -> Product1/1
  Math Function1/1 -> eta/1
  Switch2/1 -> Math Function1/2
  Product1/1 -> Switch2/2
  Constant1/1 -> Switch2/1
  Constant2/1 -> Switch2/3
  Constant/1 -> Math Function1/1
  SpdIn/1 -> Product1/2

== system EvPowertrainController3EMDualRear/Accel Pedal to Traction Wheel Torque Request/EM2WhlTrq/4EM/EMTrq2WhlTrqRear/Transmission/Diff Eta ==
  SpdIn : Inport
  TrqIn : Inport  Port=2
  Constant : Constant  Value=PlntDiffrntl2Eff
  Constant1 : Constant  SampleTime=-1
  Constant2 : Constant  Value=-1  SampleTime=-1
  Math Function1 : Math  Operator=pow  SignedPower=on  OutputSignalType=real
  Product1 : Product
  Switch2 : Switch  SaturateOnIntegerOverflow=off  InputSameDT=off
  eta : Outport  VectorParamsAs1DForOutWhenUnconnected=off
  wires:
  SpdIn/1 -> Product1/2
  Constant/1 -> Math Function1/1
  Constant2/1 -> Switch2/3
  Constant1/1 -> Switch2/1
  Product1/1 -> Switch2/2
  Switch2/1 -> Math Function1/2
  Math Function1/1 -> eta/1
  TrqIn/1 -> Product1/1

== system EvPowertrainController3EMDualRear/Accel Pedal to Traction Wheel Torque Request/EM2WhlTrq/4EM/EMTrq2WhlTrqRear/Transmission/Trans Eta ==
  TrqIn : Inport
  SpdIn : Inport  Port=2
  Gear : Inport  Port=3
  Abs1 : Abs  SaturateOnIntegerOverflow=off
  Constant : Constant  Value=PlntTransEffTempBpt(1)
  Constant1 : Constant  SampleTime=-1
  Constant2 : Constant  Value=-1  SampleTime=-1
  Eta 4D : Lookup_n-D  NumberOfTableDimensions=4  LookupTableObject=''  BreakpointsForDimension1=PlntTransEffTrqBpt  BreakpointsForDimension2=PlntTransEffSpdBpt  BreakpointsForDimension3=PlntTransGearNumVect  BreakpointsForDimension4=PlntTransEffTempBpt  Table=PlntTransEffTbl  ExtrapMethod=Clip  InternalRulePriority=Speed  RndMeth=Simplest
      settings: InputPortMap=u0,u1,u2,u3
  Math Function1 : Math  Operator=pow  SignedPower=on  OutputSignalType=real
  Product1 : Product
  Switch2 : Switch  SaturateOnIntegerOverflow=off  InputSameDT=off
  eta : Outport  VectorParamsAs1DForOutWhenUnconnected=off
  wires:
  TrqIn/1 -> Product1/1, Abs1/1
  Math Function1/1 -> eta/1
  Abs1/1 -> Eta 4D/1
  Switch2/1 -> Math Function1/2
  Product1/1 -> Switch2/2
  Constant1/1 -> Switch2/1
  Constant2/1 -> Switch2/3
  Eta 4D/1 -> Math Function1/1
  SpdIn/1 -> Product1/2, Eta 4D/2
  Gear/1 -> Eta 4D/3
  Constant/1 -> Eta 4D/4

== system EvPowertrainController3EMDualRear/Energy Management/Calculate Average EMSpd and Wheel Torque Curves for Front and Rear Axles/2EM/EMTrq2WhlTrqFrnt/Single Speed Transmission/Diff Eta ==
  note: Pwr >= 0, v = 1
      | Pwr < 0, v= -1
  SpdIn : Inport
  TrqIn : Inport  Port=2
  Constant : Constant  Value=PlntDiffrntlEff*PlntEM1TransEff
  Constant1 : Constant  SampleTime=-1
  Constant2 : Constant  Value=-1  SampleTime=-1
  Math Function1 : Math  Operator=pow  SignedPower=on  OutputSignalType=real
  Product1 : Product
  Switch2 : Switch  SaturateOnIntegerOverflow=off  InputSameDT=off
  eta : Outport  VectorParamsAs1DForOutWhenUnconnected=off
  wires:
  SpdIn/1 -> Product1/2
  Constant/1 -> Math Function1/1
  Constant2/1 -> Switch2/3
  Constant1/1 -> Switch2/1
  Product1/1 -> Switch2/2
  Switch2/1 -> Math Function1/2
  Math Function1/1 -> eta/1
  TrqIn/1 -> Product1/1

== system EvPowertrainController3EMDualRear/Energy Management/Calculate Average EMSpd and Wheel Torque Curves for Front and Rear Axles/2EM/EMTrq2WhlTrqFrnt/Transmission/Diff Eta ==
  SpdIn : Inport
  TrqIn : Inport  Port=2
  Constant : Constant  Value=PlntDiffrntlEff
  Constant1 : Constant  SampleTime=-1
  Constant2 : Constant  Value=-1  SampleTime=-1
  Math Function1 : Math  Operator=pow  SignedPower=on  OutputSignalType=real
  Product1 : Product
  Switch2 : Switch  SaturateOnIntegerOverflow=off  InputSameDT=off
  eta : Outport  VectorParamsAs1DForOutWhenUnconnected=off
  wires:
  SpdIn/1 -> Product1/2
  Constant/1 -> Math Function1/1
  Constant2/1 -> Switch2/3
  Constant1/1 -> Switch2/1
  Product1/1 -> Switch2/2
  Switch2/1 -> Math Function1/2
  Math Function1/1 -> eta/1
  TrqIn/1 -> Product1/1

== system EvPowertrainController3EMDualRear/Energy Management/Calculate Average EMSpd and Wheel Torque Curves for Front and Rear Axles/2EM/EMTrq2WhlTrqFrnt/Transmission/Trans Eta ==
  TrqIn : Inport
  SpdIn : Inport  Port=2
  Gear : Inport  Port=3
  Abs1 : Abs  SaturateOnIntegerOverflow=off
  Constant : Constant  Value=PlntTransEffTempBpt(1)
  Constant1 : Constant  SampleTime=-1
  Constant2 : Constant  Value=-1  SampleTime=-1
  Eta 4D : Lookup_n-D  NumberOfTableDimensions=4  LookupTableObject=''  BreakpointsForDimension1=PlntTransEffTrqBpt  BreakpointsForDimension2=PlntTransEffSpdBpt  BreakpointsForDimension3=PlntTransGearNumVect  BreakpointsForDimension4=PlntTransEffTempBpt  Table=PlntTransEffTbl  ExtrapMethod=Clip  InternalRulePriority=Speed  RndMeth=Simplest
      settings: InputPortMap=u0,u1,u2,u3
  Math Function1 : Math  Operator=pow  SignedPower=on  OutputSignalType=real
  Product1 : Product
  Switch2 : Switch  SaturateOnIntegerOverflow=off  InputSameDT=off
  eta : Outport  VectorParamsAs1DForOutWhenUnconnected=off
  wires:
  TrqIn/1 -> Product1/1, Abs1/1
  Math Function1/1 -> eta/1
  Abs1/1 -> Eta 4D/1
  Switch2/1 -> Math Function1/2
  Product1/1 -> Switch2/2
  Constant1/1 -> Switch2/1
  Constant2/1 -> Switch2/3
  Eta 4D/1 -> Math Function1/1
  SpdIn/1 -> Product1/2, Eta 4D/2
  Gear/1 -> Eta 4D/3
  Constant/1 -> Eta 4D/4
